simulink model "trms_paper_simulink_pd_varying_plant"  (R2024a)
settings: Solver=VariableStepAuto  StartTime=0.0  StopTime=1000  RelTol=1e-9
values from neighbouring files (symbols this model uses):
  Am = [0     1     0     0 ... (first row only)    [trms_paper.m]
  Bm = [0    0 ... (first row only)    [trms_paper.m]
  S = GammaK*B0a'*P    [trms_paper.m]
settings Model: Creator=Unnati  LastModifiedBy=Unnati

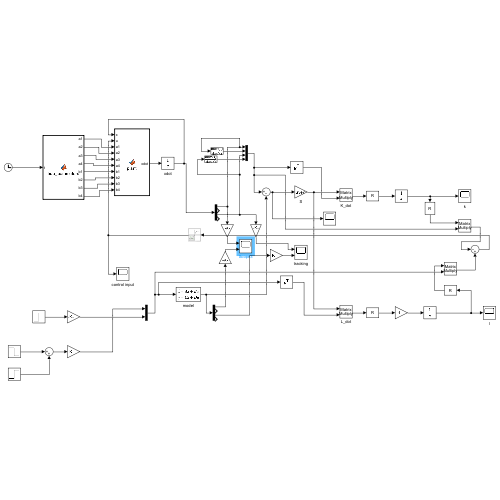
[thumbnail: Simulink's stored preview of the top-level diagram]
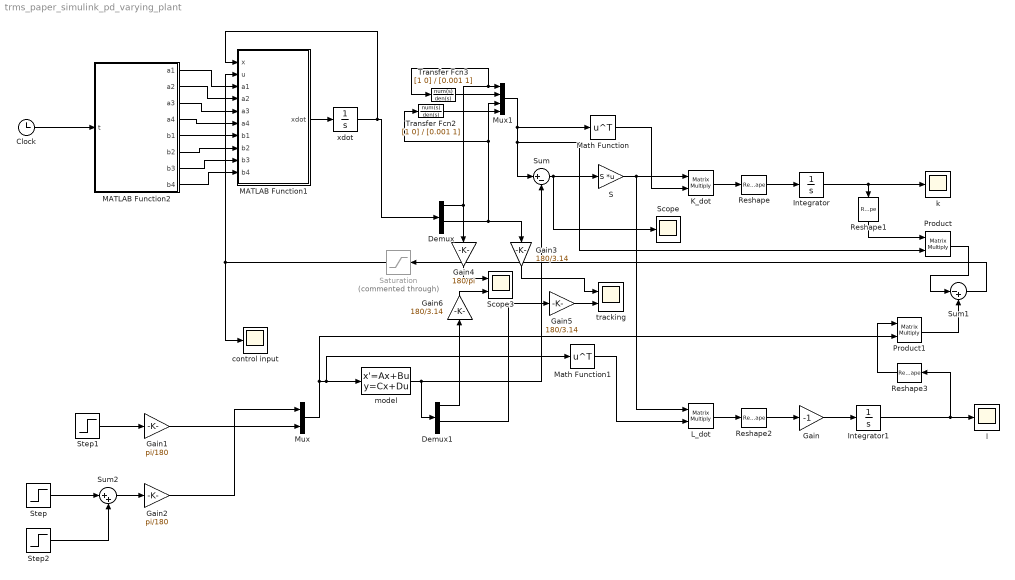
== system trms_paper_simulink_pd_varying_plant ==
  Clock : Clock
  Demux : Demux
  Demux1 : Demux
  Gain : Gain  Gain=-1
  Gain1 : Gain  Gain=pi/180
  Gain2 : Gain  Gain=pi/180
  Gain3 : Gain  Gain=180/3.14
  Gain4 : Gain  Gain=180/pi
  Gain5 : Gain  Gain=180/3.14
  Gain6 : Gain  Gain=180/3.14
  Integrator : Integrator
  Integrator1 : Integrator
  K_dot : Product  Multiplication=Matrix(*)
  L_dot : Product  Multiplication=Matrix(*)
  MATLAB Function1 : MATLAB Function  TreatAsAtomicUnit=on
  MATLAB Function2 : MATLAB Function  TreatAsAtomicUnit=on
  Math Function : Math  Operator=transpose
  Math Function1 : Math  Operator=transpose
  Mux : Mux  Inputs=2
  Mux1 : Mux
  Product : Product  Multiplication=Matrix(*)
  Product1 : Product  Multiplication=Matrix(*)
  Reshape : Reshape  OutputDimensionality=Customize  OutputDimensions=[8,1]
  Reshape1 : Reshape  OutputDimensionality=Customize  OutputDimensions=[2,4]
  Reshape2 : Reshape  OutputDimensionality=Customize  OutputDimensions=[4,1]
  Reshape3 : Reshape  OutputDimensionality=Customize  OutputDimensions=[2,2]
  S : Gain  Gain=S  Multiplication=Matrix(K*u) (u vector)
  Saturation : Saturate  Commented=through  UpperLimit=24  LowerLimit=-24
  Scope : Scope
  Scope3 : Scope  NumInputPorts=2
  Step : Step  Time=600  Before=10  After=0  SampleTime=0
  Step1 : Step  After=10  SampleTime=0
  Step2 : Step  Time=800  After=10  SampleTime=0
  Sum : Sum  Inputs=|+-
  Sum1 : Sum  Inputs=|-+
  Sum2 : Sum  Inputs=|++
  Transfer Fcn2 : TransferFcn  Numerator=[1 0]  Denominator=[0.001 1]
  Transfer Fcn3 : TransferFcn  Numerator=[1 0]  Denominator=[0.001 1]
  control input : Scope
  k : Scope
  l : Scope
  model : StateSpace  A=Am  B=Bm  C=eye(4)  D=[0 0;0 0;0 0;0 0]  InitialCondition=0
  tracking : Scope  NumInputPorts=2
  xdot : Integrator
  wires:
  Mux1/1 -> Product/2, Sum/1, Math Function/1
  Reshape2/1 -> Gain/1
  Step1/1 -> Gain1/1
  Demux/1 -> Transfer Fcn3/1, Mux1/1, Gain4/1
  Transfer Fcn2/1 -> Mux1/4
  Gain4/1 -> Scope3/1
  Integrator/1 -> k/1, Reshape1/1
  Gain1/1 -> Mux/2
  Integrator1/1 -> Reshape3/1, l/1
  Reshape3/1 -> Product1/1
  S/1 -> L_dot/1, K_dot/1
  Demux/3 -> Gain3/1, Mux1/3, Transfer Fcn2/1
  Saturation/1 -> MATLAB Function1/2(u), control input/1
  Gain3/1 -> tracking/1
  Gain2/1 -> Mux/1
  Transfer Fcn3/1 -> Mux1/2
  Gain/1 -> Integrator1/1
  Reshape/1 -> Integrator/1
  Sum1/1 -> Saturation/1
  Reshape1/1 -> Product/1
  Gain6/1 -> Scope3/2
  Demux1/1 -> Gain6/1
  Mux/1 -> Product1/2, Math Function1/1, model/1
  Product1/1 -> Sum1/2
  L_dot/1 -> Reshape2/1
  Product/1 -> Sum1/1
  K_dot/1 -> Reshape/1
  model/1 -> Demux1/1, Sum/2
  Math Function1/1 -> L_dot/2
  xdot/1 -> MATLAB Function1/1(x), Demux/1
  Demux1/3 -> Gain5/1
  Gain5/1 -> tracking/2
  Math Function/1 -> K_dot/2
  Sum/1 -> Scope/1, S/1
  Clock/1 -> MATLAB Function2/1("t ")
  MATLAB Function2/1(a1) -> MATLAB Function1/3(a1)
  MATLAB Function2/2(a2) -> MATLAB Function1/4(a2)
  MATLAB Function2/3(a3) -> MATLAB Function1/5(a3)
  MATLAB Function2/4(a4) -> MATLAB Function1/6(a4)
  MATLAB Function2/5(b1) -> MATLAB Function1/7(b1)
  MATLAB Function2/6(b2) -> MATLAB Function1/8(b2)
  MATLAB Function2/7(b3) -> MATLAB Function1/9(b3)
  MATLAB Function2/8(b4) -> MATLAB Function1/10(b4)
  MATLAB Function1/1(xdot) -> xdot/1
  Sum2/1 -> Gain2/1
  Step/1 -> Sum2/1
  Step2/1 -> Sum2/2

== matlab function trms_paper_simulink_pd_varying_plant/MATLAB Function1 ==
  data: x input; u input; xdot output; a1 input; a2 input; a3 input; a4 input; b1 input; b2 input; b3 input; b4 input
function xdot = plant(x,u,a1,a2,a3,a4,b1,b2,b3,b4)

xdot = zeros(4,1);

xdot(1) = x(2);

xdot(2) = -a1*x(1) - a2*x(2) ...
          + b1*u(1) + b2*u(2);

xdot(3) = x(4);

xdot(4) = -a3*x(3) - a4*x(4) ...
          + b3*u(1) + b4*u(2);

end

== matlab function trms_paper_simulink_pd_varying_plant/MATLAB Function2 ==
  data: t input; a1 output; a2 output; a3 output; a4 output; b1 output; b2 output; b3 output; b4 output
function [a1,a2,a3,a4,b1,b2,b3,b4] = true_parameters(t)

% Nominal true parameters
a1_nom = 1.71;
a2_nom = 0.32;
a3_nom = 0;
a4_nom = 1;

b1_nom = 0.05;
b2_nom = 0.095;
b3_nom = -0.12;
b4_nom = 0.1;

if t < 500

    a1 = a1_nom;
    a2 = a2_nom;
    a3 = a3_nom;
    a4 = a4_nom;

    b1 = b1_nom;
    b2 = b2_nom;
    b3 = b3_nom;
    b4 = b4_nom;

else

    a1 = 1.20*a1_nom;
    a2 = 1.20*a2_nom;
    a3 = 1.20*a3_nom;
    a4 = 1.20*a4_nom;

    b1 = 1.2*b1_nom;
    b2 = 1.2*b2_nom;
    b3 = 1.2*b3_nom;
    b4 = 1.2*b4_nom;

end
